simulink model "VINS"  (R2018a)
settings: Solver=FixedStepDiscrete  StartTime=0.0  StopTime=inf  FixedStep=1/Fs  RelTol=1e-3  EnableMultiTasking=on
PreLoadFcn:
  | modelDef = getModelDef(calibrateSFMA);
  | 
  | %imuPar = getImuPar('lmvpUncalibrated');
  | 
  | timeMatchThreshold = 1000;
undefined symbols (not defined in the file or in its folder): beep, dejitter_on, Fs, homogeneous3x4Transform_k_kmin1, imuLocationMm, imuPar, numStates, simData, tstamp_k_us, tstamp_kmin1_us
libraries: simulink x69, dspmtrx3 x35, dspindex x9, vrlib x7, dspstat3 x7, dspinverses x6, dspsigops x5, dspmathops x2, rtwdemowidgets x1, dspfactors x1, simulink_extras x1
(part 3 of 6)

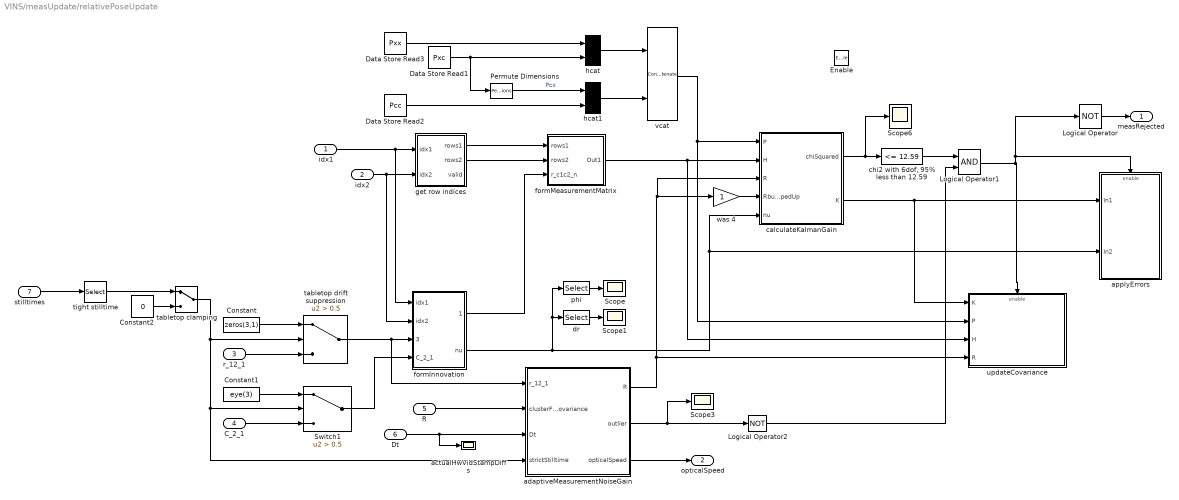
== system VINS/measUpdate/relativePoseUpdate ==
  idx1 : Inport
  idx2 : Inport  Port=2
  r_12_1 : Inport  Port=3
  C_2_1 : Inport  Port=4
  R : Inport  Port=5
  Dt : Inport  Port=6
  stilltimes : Inport  Port=7
  Enable : EnablePort
  Constant : Constant  Value=zeros(3,1)  OutDataTypeStr=Inherit: Inherit via back propagation
  Constant1 : Constant  Value=eye(3)  OutDataTypeStr=Inherit: Inherit via back propagation
  Constant2 : Constant  Value=0
  Data Store Read1 : DataStoreRead  DataStoreName=Pxc
  Data Store Read2 : DataStoreRead  DataStoreName=Pcc
  Data Store Read3 : DataStoreRead  DataStoreName=Pxx
  Logical Operator : Logic  Operator=NOT  Inputs=1  IconShape=distinctive  AllPortsSameDT=off  OutDataTypeStr=boolean
  Logical Operator1 : Logic  AllPortsSameDT=off  OutDataTypeStr=boolean
  Logical Operator2 : Logic  Operator=NOT  Inputs=1  IconShape=distinctive  AllPortsSameDT=off  OutDataTypeStr=boolean
  Permute Dimensions : PermuteDimensions
  Scope{,1,3,6} (4 alike) : Scope
  Switch1 : Switch  Criteria=u2 > Threshold  Threshold=0.5
  actualHwVidStampDiffs : Scope
  adaptiveMeasurementNoiseGain : Subsystem  TreatAsAtomicUnit=on
      settings: RTWSystemCode=Nonreusable function  RTWFcnNameOpts=Use subsystem name
  applyErrors : Subsystem
      settings: RTWSystemCode=Nonreusable function  RTWFcnNameOpts=Use subsystem name
  calculateKalmanGain : MATLAB Function  TreatAsAtomicUnit=on
  "chi2 with 6dof, 95% less than 12.59" : simulink/Logic and Bit Operations/Compare To Constant  relop=<=  const=12.59  OutDataTypeStr=boolean
  dr : Selector  InputPortWidth=6  IndexOptions=Index vector (dialog)  Indices=[4 5 6]  OutputSizes=1
  formInnovation : Subsystem  TreatAsAtomicUnit=on
  formMeasurementMatrix : Subsystem
  get row indices : Subsystem  TreatAsAtomicUnit=on
  hcat : Concatenate  Mode=Multidimensional array  ConcatenateDimension=2
  hcat1 : Concatenate  Mode=Multidimensional array  ConcatenateDimension=2
  phi : Selector  InputPortWidth=6  IndexOptions=Index vector (dialog)  Indices=[1 2 3]  OutputSizes=1
  tabletop clamping : ManualSwitch
  tabletop drift suppression : Switch  Criteria=u2 > Threshold  Threshold=0.5
  tight stilltime : Selector  InputPortWidth=2  IndexOptions=Index vector (dialog)  Indices=1  OutputSizes=1
  updateCovariance : Subsystem
  vcat : Concatenate  Mode=Multidimensional array
  was 4 : Gain  OutDataTypeStr=Inherit: Inherit via back propagation
  measRejected : Outport  OutputWhenDisabled=reset  InitialOutput=0
  opticalSpeed : Outport  Port=2  InitialOutput=100
  wires:
  calculateKalmanGain/2(K) -> updateCovariance/1(K), applyErrors/1(In1)
  vcat/1 -> updateCovariance/2(P), calculateKalmanGain/1(P)
  tabletop drift suppression/1 -> adaptiveMeasurementNoiseGain/1(r_12_1), formInnovation/3(r_c1c2_c1)
  idx1/1 -> formInnovation/1(idx1), get row indices/1(idx1)
  idx2/1 -> formInnovation/2(idx2), get row indices/2(idx2)
  formInnovation/2(nu) -> calculateKalmanGain/5(nu), applyErrors/2(In2), phi/1, dr/1
  formMeasurementMatrix/1(Out1) -> updateCovariance/3(H), calculateKalmanGain/2(H)
  get row indices/1(rows1) -> formMeasurementMatrix/1(rows1)
  get row indices/2(rows2) -> formMeasurementMatrix/2(rows2)
  hcat/1 -> vcat/1
  hcat1/1 -> vcat/2
  Data Store Read3/1 -> hcat/1
  Data Store Read1/1 -> Permute Dimensions/1, hcat/2
  Permute Dimensions/1 -> hcat1/1  "Pcx"
  Data Store Read2/1 -> hcat1/2
  formInnovation/1(r_c1c2_n) -> formMeasurementMatrix/3(r_c1c2_n)
  phi/1 -> Scope/1
  dr/1 -> Scope1/1
  calculateKalmanGain/1(chiSquared) -> "chi2 with 6dof, 95% less than 12.59"/1, Scope6/1
  Logical Operator1/1 -> updateCovariance/Enable, Logical Operator/1, applyErrors/Enable
  Logical Operator/1 -> measRejected/1
  was 4/1 -> calculateKalmanGain/4(RbumpedUp)
  Switch1/1 -> formInnovation/4(C_2_1)
  "chi2 with 6dof, 95% less than 12.59"/1 -> Logical Operator1/1
  R/1 -> adaptiveMeasurementNoiseGain/2(clusterFlowCovariance)
  adaptiveMeasurementNoiseGain/1(R) -> updateCovariance/4(R), calculateKalmanGain/3(R), was 4/1
  adaptiveMeasurementNoiseGain/2(outlier) -> Scope3/1, Logical Operator2/1
  Logical Operator2/1 -> Logical Operator1/2
  Dt/1 -> actualHwVidStampDiffs/1, adaptiveMeasurementNoiseGain/3(Dt)
  C_2_1/1 -> Switch1/3
  r_12_1/1 -> tabletop drift suppression/3
  Constant/1 -> tabletop drift suppression/1
  Constant1/1 -> Switch1/1
  stilltimes/1 -> tight stilltime/1
  tabletop clamping/1 -> tabletop drift suppression/2, adaptiveMeasurementNoiseGain/4(strictStilltime), Switch1/2
  tight stilltime/1 -> tabletop clamping/1
  Constant2/1 -> tabletop clamping/2
  adaptiveMeasurementNoiseGain/3(opticalSpeed) -> opticalSpeed/1

== system VINS/measUpdate/relocalize ==
  note: Absolute Pose Update should trigger relocalization if:
      |      * APU position is > __ cm away from current nav position
      |      * APU heading is > __ mrad away from current naw heading
      |      * current position uncertainty is > __
      |      * current heading uncertainty is > __
      |      * this is the first APU (do we need this?)
  innovation : Inport
  APU : Inport  Port=2
  Bus Selector : BusSelector  OutputSignals=doAbsolutePoseUpdate,r_nb_n,C_b_n
  Subsystem : Subsystem
  reloc : Outport
  wires:
  APU/1 -> Bus Selector/1
  Bus Selector/1 -> Subsystem/Enable  "<doAbsolutePoseUpdate>"
  Bus Selector/2 -> Subsystem/1(r_nc_n)  "<r_nb_n>"
  Bus Selector/3 -> Subsystem/2(<C_b_n>)  "<C_b_n>"
  innovation/1 -> Subsystem/3(innovation)
  Subsystem/1(reloc) -> reloc/1

== system VINS/measUpdate/wipe out delayed states ==
  note: wiping out tstamp_list should be sufficient to cause delayed states in buffers to be ignored
  Enable : EnablePort  ShowOutputPort=on
  Data Store Write5 : DataStoreWrite  DataStoreName=tstamp_list
  Ground : Ground
  setP : Subsystem
  wires:
  Ground/1 -> Data Store Write5/1
  Enable/1 -> setP/Enable

== system VINS/measUpdate/zuptMeasUpdate ==
  stilltime : Inport
  Enable : EnablePort
  0.01s to 10s : Saturate  UpperLimit=10  LowerLimit=0.01
  Constant : Constant  Value=eye(3)  OutDataTypeStr=Inherit: Inherit via back propagation
  Constant1 : Constant  Value=eye(3)  OutDataTypeStr=Inherit: Inherit via back propagation
  Constant2 : Constant  Value=zeros(3,9)  VectorParams1D=off  OutDataTypeStr=Inherit: Inherit via back propagation
  Constant3 : Constant  Value=zeros(3,1)  VectorParams1D=off  OutDataTypeStr=Inherit: Inherit via back propagation
  DT police : Subsystem  TreatAsAtomicUnit=on
  DT police1 : Subsystem  TreatAsAtomicUnit=on
  Data Store Read1 : DataStoreRead  DataStoreName=vnav
  Data Store Read3 : DataStoreRead  DataStoreName=Pxx
  Data Store Write : DataStoreWrite  DataStoreName=Pxx
  Math Function : Math  Operator=reciprocal  SaturateOnIntegerOverflow=on
  Math Function1 : Math  Operator=square  SaturateOnIntegerOverflow=on
  Matrix Concatenate : Concatenate  Mode=Multidimensional array  ConcatenateDimension=2
  Pad : dspsigops/Pad  padAlong=Rows  dimsToPad=1  valSrc=Specify via dialog  padVal=0  spec=Output size  padNumOutRowsSpecMethod=User-specified  numOutRows=1  padNumOutColsSpecMethod=User-specified  numOutCols=modelDef.numStates  isVarDimsMode=off  padBeginning=0  padEnd=0  outSizeMode=User-specified  outSize=1  padSigAt=End  trunc_flag=None  roundingMode=Floor  overflowMode=off  truncOrWrapMode=Truncate  wrap_flag=None
      settings: SourceProductName=DSP System Toolbox  SourceProductBaseCode=DS
  Product1 : Product  Multiplication=Matrix(*)
  Product2 : Product
  Saturation : Saturate  UpperLimit=100  LowerLimit=0.1
  Scope : Scope
  Scope1 : Scope
  Selector : Selector  InputPortWidth=2  IndexOptions=Index vector (dialog)  Indices=2  OutputSizes=1
  Sum1 : Sum  Inputs=|+-
  applyErrors : Subsystem
  calculateKalmanGain : MATLAB Function  TreatAsAtomicUnit=on
  josephCovarianceUpdate : MATLAB Function  TreatAsAtomicUnit=on
  wires:
  Constant3/1 -> Sum1/2
  Data Store Read1/1 -> Sum1/1
  0.01s to 10s/1 -> Math Function/1
  Constant1/1 -> Matrix Concatenate/2
  Constant2/1 -> Matrix Concatenate/1
  Sum1/1 -> Product1/2, Scope1/1  "nu = dv = vhat - vtrue"
  josephCovarianceUpdate/1(Pplus) -> Data Store Write/1
  Matrix Concatenate/1 -> Pad/1
  Data Store Read3/1 -> josephCovarianceUpdate/1(P), calculateKalmanGain/1(P)
  Product2/1 -> DT police1/1(In1), josephCovarianceUpdate/4(R), calculateKalmanGain/3(R)
  Product1/1 -> applyErrors/1(errorStateEstimates)  "errors"
  Constant/1 -> Product2/1
  Math Function/1 -> Saturation/1
  Saturation/1 -> Math Function1/1, Scope/1
  stilltime/1 -> Selector/1
  Math Function1/1 -> Product2/2
  Pad/1 -> DT police/1(In1), josephCovarianceUpdate/3(H), calculateKalmanGain/2(H)
  calculateKalmanGain/2(K) -> josephCovarianceUpdate/2(K), Product1/1
  Selector/1 -> 0.01s to 10s/1

== system VINS/reportOutputs/dejitter ==
  note: Velocity of corrections should be limited to 10% of the
      | optical velocity when confident optical velocity exists.
      |
      | However, to prevent unbounded drift,  increase the correction factor if the error gets very large.
  r_jit : Inport
  v : Inport  Port=2
  opticalSpeed : Inport  Port=3
  Dt : Inport  Port=4
  reloc : Inport  Port=5
  1-D Lookup Table : Lookup_n-D  NumberOfTableDimensions=1  BreakpointsForDimension1="[0  0.005 0.01 0.02 0.03 0.04]"  Table="[0    0.02   0.08    0.2       1      1]"  InternalRulePriority=Speed  RndMeth=Simplest  InputSameDT=on
  1-D Lookup Table1 : Lookup_n-D  Commented=on  NumberOfTableDimensions=1  BreakpointsForDimension1="[0  0.05 0.1 0.2 0.3 0.4]"  Table="[0.002    0.02   0.08    0.2       1      1]*0.1"  InternalRulePriority=Speed  RndMeth=Simplest  InputSameDT=on
  Gain : Gain  Gain=1/2
  Gain1 : Gain  Gain=0.1
  Math Function : Math  Operator=square  SaturateOnIntegerOverflow=on
  Math Function1 : Math  Operator=square  SaturateOnIntegerOverflow=on
  MinMax : MinMax  Function=max  Inputs=2
  Product : Product
  Product1 : Product
  Product2 : Product
  Scope1 : Scope  NumInputPorts=2
  Scope2 : Scope
  Scope3 : Scope
  Sqrt : Sqrt  SaturateOnIntegerOverflow=on
  Sqrt1 : Sqrt  SaturateOnIntegerOverflow=on
  Sum : Sum  Inputs=|++
  Sum1 : Sum
  Sum2 : Sum  Inputs=|+-
  Sum3 : Sum  Inputs=|++
  Sum4 : Sum  Inputs=+
  Sum5 : Sum  Inputs=+
  midpoint velocity : Delay  DelayLength=1  InitialConditionSource=Input port
      settings: InputPortMap=u0,p4
  position integrator : Delay  DelayLength=1  InitialConditionSource=Input port  ExternalReset=Level
      settings: InputPortMap=u0,r5,p4
  r_clean : Outport
  wires:
  position integrator/1 -> Sum1/2
  r_jit/1 -> Sum2/1, position integrator/3  "measPos"
  v/1 -> Sum/1, midpoint velocity/2, midpoint velocity/1
  midpoint velocity/1 -> Sum/2
  Sum/1 -> Gain/1
  Gain/1 -> Product/1, Math Function1/1
  Product/1 -> Sum1/1
  Sum1/1 -> Sum3/2, Sum2/2  "predPos"
  Sum2/1 -> Math Function/1, Product1/2  "innov"
  Product1/1 -> Sum3/1
  Sum3/1 -> position integrator/1, r_clean/1
  Math Function/1 -> Sum4/1
  Sum4/1 -> Sqrt/1
  Sqrt/1 -> 1-D Lookup Table/1, Product2/2  "needed delta_r"
  MinMax/1 -> Product1/1, Scope3/1  "jitter fraction"
  Sum5/1 -> Sqrt1/1
  Math Function1/1 -> Sum5/1
  Sqrt1/1 -> Scope1/2, 1-D Lookup Table1/1, Gain1/1  "INS speed"
  reloc/1 -> position integrator/2
  Gain1/1 -> MinMax/1
  Product2/1 -> Scope2/1, MinMax/2
  1-D Lookup Table/1 -> Product2/1
  Dt/1 -> Product/2
  opticalSpeed/1 -> Scope1/1

== system VINS/reportOutputs/updateDistTravelled ==
  pos : Inport
  Compare To Constant : simulink/Logic and Bit Operations/Compare To Constant  relop=>=  const=0.003  OutDataTypeStr=boolean
  Compare To Zero : simulink/Logic and Bit Operations/Compare To Zero  relop===  OutDataTypeStr=boolean
  Data Store Read : DataStoreRead  DataStoreName=distTravelled
  Logical Operator : Logic  Operator=OR  AllPortsSameDT=off  OutDataTypeStr=boolean
  Math Function : Math  Operator=square  SaturateOnIntegerOverflow=on
  Sqrt : Sqrt  SaturateOnIntegerOverflow=on
  Sum2 : Sum  Inputs=|+-
  Sum4 : Sum  Inputs=+
  Unit Delay : UnitDelay  SampleTime=-1
  increment distTravelled : Subsystem  TreatAsAtomicUnit=on
  latch : Subsystem  TreatAsAtomicUnit=on
  reset occured : simulink/Logic and Bit Operations/Detect Rise Positive  vinit=0  OutDataTypeStr=boolean
  distTravelled : Outport
  wires:
  pos/1 -> Sum2/1, latch/1(In1)  "measPos"
  latch/1(Out1) -> Sum2/2  "predPos"
  Sum2/1 -> Math Function/1  "innov"
  Math Function/1 -> Sum4/1
  Sum4/1 -> Sqrt/1
  Sqrt/1 -> increment distTravelled/1(deltaPos), Compare To Constant/1  "position change"
  Data Store Read/1 -> Compare To Zero/1
  Compare To Zero/1 -> reset occured/1
  reset occured/1 -> Logical Operator/2
  Compare To Constant/1 -> Unit Delay/1, increment distTravelled/Enable
  increment distTravelled/1(distTravelled) -> distTravelled/1
  Logical Operator/1 -> latch/Enable
  Unit Delay/1 -> Logical Operator/1

== system VINS/sensorCompensation/DT police ==
  In1 : Inport
  Data Store Read : DataStoreRead  DataStoreName=DataTypeRef
  Data Type Duplicate : DataTypeDuplicate
  wires:
  Data Store Read/1 -> Data Type Duplicate/1
  In1/1 -> Data Type Duplicate/2

== system VINS/sensorCompensation/DT police1 ==
  In1 : Inport
  Data Store Read : DataStoreRead  DataStoreName=DataTypeRef
  Data Type Duplicate : DataTypeDuplicate
  wires:
  In1/1 -> Data Type Duplicate/2
  Data Store Read/1 -> Data Type Duplicate/1

== system VINS/sensorCompensation/detectAccelSaturation ==
  In1 : Inport
  Abs : Abs
  Abs1 : Abs
  Abs2 : Abs
  Compare To Constant : simulink/Logic and Bit Operations/Compare To Constant  relop=>  const=39  OutDataTypeStr=boolean
  Compare To Constant1 : simulink/Logic and Bit Operations/Compare To Constant  relop=<  const=0.002  OutDataTypeStr=boolean
  Compare To Constant2 : simulink/Logic and Bit Operations/Compare To Constant  relop=<  const=0.002  OutDataTypeStr=boolean
  Logical Operator : Logic  Inputs=3  AllPortsSameDT=off  OutDataTypeStr=boolean
  Logical Operator1 : Logic  Operator=OR  Inputs=1  AllPortsSameDT=off  OutDataTypeStr=boolean
  Logical Operator2 : Logic  AllPortsSameDT=off  OutDataTypeStr=boolean
  Logical Operator3 : Logic  AllPortsSameDT=off  OutDataTypeStr=boolean
  Scope : Scope
  Scope1 : Scope
  Scope2 : Scope
  Sum1 : Sum  Inputs=+-|
  Sum2 : Sum  Inputs=+-|
  Unit Delay{,1..3} (4 alike) : UnitDelay  SampleTime=-1
  set 0x01 bit : Subsystem  TreatAsAtomicUnit=on
  wires:
  Logical Operator/1 -> Scope/1, Logical Operator3/1
  Unit Delay1/1 -> Logical Operator/3
  Unit Delay/1 -> Logical Operator/2, Unit Delay1/1
  Compare To Constant/1 -> Logical Operator/1, Unit Delay/1
  Abs/1 -> Compare To Constant/1
  In1/1 -> Sum1/2, Unit Delay2/1, Abs/1
  Sum2/1 -> Abs1/1
  Sum1/1 -> Abs2/1
  Abs1/1 -> Compare To Constant1/1
  Abs2/1 -> Compare To Constant2/1
  Logical Operator2/1 -> Scope1/1, Logical Operator3/2
  Logical Operator3/1 -> Logical Operator1/1
  Logical Operator1/1 -> Scope2/1, set 0x01 bit/Enable
  Unit Delay2/1 -> Unit Delay3/1, Sum2/2, Sum1/1
  Unit Delay3/1 -> Sum2/1
  Compare To Constant1/1 -> Logical Operator2/1
  Compare To Constant2/1 -> Logical Operator2/2

== system VINS/sensorCompensation/detectGyroSaturation ==
  In1 : Inport
  Abs : Abs
  Compare To Constant : simulink/Logic and Bit Operations/Compare To Constant  relop=>  const=1900*pi/180  OutDataTypeStr=boolean
  Logical Operator : Logic  Inputs=3  AllPortsSameDT=off  OutDataTypeStr=boolean
  Logical Operator1 : Logic  Operator=OR  Inputs=1  AllPortsSameDT=off  OutDataTypeStr=boolean
  Unit Delay : UnitDelay  SampleTime=-1
  Unit Delay1 : UnitDelay  SampleTime=-1
  set 0x02 bit : Subsystem  TreatAsAtomicUnit=on
  wires:
  In1/1 -> Abs/1
  Abs/1 -> Compare To Constant/1
  Compare To Constant/1 -> Unit Delay/1, Logical Operator/1
  Unit Delay/1 -> Unit Delay1/1, Logical Operator/2
  Unit Delay1/1 -> Logical Operator/3
  Logical Operator/1 -> Logical Operator1/1
  Logical Operator1/1 -> set 0x02 bit/Enable

== system VINS/sensorCompensation/set 0x04 bit ==
  Enable : EnablePort
  Assertion : Assertion  StopWhenAssertionFail=off
  Bit Set : simulink/Logic and Bit Operations/Bit Set  iBit=2
      settings: SourceProductName=Simulink  SourceProductBaseCode=SL
  Constant : Constant  Value=false
  Data Store Read : DataStoreRead  DataStoreName=errorBitfield
  Data Store Write : DataStoreWrite  DataStoreName=errorBitfield
  wires:
  Data Store Read/1 -> Bit Set/1
  Bit Set/1 -> Data Store Write/1
  Constant/1 -> Assertion/1

== system VINS/stilltimes/DT police ==
  In1 : Inport
  Data Store Read : DataStoreRead  DataStoreName=DataTypeRef
  Data Type Duplicate : DataTypeDuplicate
  wires:
  Data Store Read/1 -> Data Type Duplicate/1
  In1/1 -> Data Type Duplicate/2

== system VINS/stilltimes/DT police1 ==
  In1 : Inport
  Data Store Read : DataStoreRead  DataStoreName=DataTypeRef
  Data Type Duplicate : DataTypeDuplicate
  wires:
  In1/1 -> Data Type Duplicate/2
  Data Store Read/1 -> Data Type Duplicate/1

== system VINS/uncomment and set zero noise for verification/compare  timestamps ==
  t1_meas : Inport
  t1_pred : Inport  Port=2
  t2_meas : Inport  Port=3
  t2_pred : Inport  Port=4
  Enable : EnablePort
  Assertion : Assertion  Commented=on
  Assertion1 : Assertion  Commented=on
  Compare To Constant : simulink/Logic and Bit Operations/Compare To Constant  relop=<=  const=3.0  OutDataTypeStr=boolean
  Compare To Constant1 : simulink/Logic and Bit Operations/Compare To Constant  relop=<=  const=3.0  OutDataTypeStr=boolean
  Scope : Scope
  Scope1 : Scope
  Scope2 : Scope
  Sum : Sum  Inputs=|+-
  Sum1 : Sum  Inputs=|+-
  Sum2 : Sum  Inputs=|+-
  Unit Delay : UnitDelay  SampleTime=-1
  wires:
  Sum/1 -> Compare To Constant/1, Scope/1
  t1_meas/1 -> Sum2/1, Sum/1
  t2_meas/1 -> Unit Delay/1, Sum1/1
  Sum1/1 -> Compare To Constant1/1, Scope1/1
  t1_pred/1 -> Sum/2
  t2_pred/1 -> Sum1/2
  Compare To Constant/1 -> Assertion/1
  Compare To Constant1/1 -> Assertion1/1
  Unit Delay/1 -> Sum2/2
  Sum2/1 -> Scope2/1

== system VINS/uncomment and set zero noise for verification/initialize H ==
  Enable : EnablePort
  Constant : Constant  Value=[0 0 0 1]  VectorParams1D=off  OutDataTypeStr=Inherit: Inherit via back propagation
  Constant9 : Constant  Value=imuLocationMm  OutDataTypeStr=Inherit: Inherit via back propagation
  Data Store Read : DataStoreRead  DataStoreName=Cbn
  Data Store Read1 : DataStoreRead  DataStoreName=rnav
  Data Store Write : DataStoreWrite  DataStoreName=H
  Gain : Gain  Gain=1/1000
  Matrix Concatenate : Concatenate  Mode=Multidimensional array  ConcatenateDimension=2
  Matrix Concatenate1 : Concatenate  Mode=Multidimensional array
  Matrix Multiply : Product  Multiplication=Matrix(*)
  Sum : Sum  Inputs=-+|
  wires:
  Constant/1 -> Matrix Concatenate1/2
  Sum/1 -> Matrix Concatenate/2  "r_nc_n"
  Matrix Concatenate/1 -> Matrix Concatenate1/1
  Matrix Concatenate1/1 -> Data Store Write/1
  Data Store Read1/1 -> Sum/2  "r_nb_n"
  Constant9/1 -> Gain/1
  Matrix Multiply/1 -> Sum/1  "r_cb_n"
  Data Store Read/1 -> Matrix Multiply/1, Matrix Concatenate/1  "Ccn = Cbn"
  Gain/1 -> Matrix Multiply/2  "r_cb_c"

== system VINS/uncomment and set zero noise for verification/latch ==
  r_12_1 : Inport
  C_2_1 : Inport  Port=2
  t1 : Inport  Port=3
  t2 : Inport  Port=4
  delayFrames : Inport  Port=5
  Enable : EnablePort
  Delay{,1..3} (4 alike) : Delay  DelayLengthSource=Input port
      settings: InputPortMap=u0,p1
  r21 : Outport
  C21 : Outport  Port=2
  tout1 : Outport  Port=3
  tout2 : Outport  Port=4
  wires:
  r_12_1/1 -> Delay/1
  C_2_1/1 -> Delay1/1
  t1/1 -> Delay2/1
  t2/1 -> Delay3/1
  Delay/1 -> r21/1
  Delay1/1 -> C21/1
  Delay2/1 -> tout1/1
  Delay3/1 -> tout2/1
  delayFrames/1 -> Delay3/2, Delay2/2, Delay1/2, Delay/2

== system VINS/uncomment and set zero noise for verification/plot errors ==
  dr_meas : Inport
  C21_meas : Inport  Port=2
  dr_pred : Inport  Port=3
  C21_pred : Inport  Port=4
  Enable : EnablePort
  Cumulative Sum : dspmathops/Cumulative Sum  dim=Channels (running sum)  reset_popup=None  roundingMode=Floor  overflowMode=off  outputDataTypeStr=Inherit: Same as accumulator  outputMin=[]  outputMax=[]  outputLastDataTypeStr=Inherit: Same as accumulator
      settings: SourceProductName=DSP System Toolbox
  Cumulative Sum1 : dspmathops/Cumulative Sum  dim=Channels (running sum)  reset_popup=None  roundingMode=Floor  overflowMode=off  outputDataTypeStr=Inherit: Same as accumulator  outputMin=[]  outputMax=[]  outputLastDataTypeStr=Inherit: Same as accumulator
      settings: SourceProductName=DSP System Toolbox
  MATLAB Function1 : MATLAB Function  TreatAsAtomicUnit=on
  MATLAB Function2 : MATLAB Function  TreatAsAtomicUnit=on
  MATLAB Function3 : MATLAB Function  TreatAsAtomicUnit=on
  Matrix Multiply : Product  Multiplication=Matrix(*)
  Permute Dimensions : PermuteDimensions
  Reshape : Reshape
  Scope{,1..2,5..6} (5 alike) : Scope
  Scope3 : Scope  NumInputPorts=2
  Scope4 : Scope  NumInputPorts=2
  Sum : Sum  Inputs=|+-
  det3x3 : Fcn  Expr=|
      | u(1)*
      | (u(5)*u(9) - u(8)*u(6)
      | ) - u(4)*
      | (u(2)*
      | u(9) - u(8)*u(3)
      | ) + u(7)*
      | (u(2)*u(6) - u(5)*u(3)
      | )
  deul_meas : Outport
  deul_pred : Outport  Port=2
  drmeas : Outport  Port=3
  drpred : Outport  Port=4
  wires:
  dr_meas/1 -> drmeas/1, Scope4/1, Cumulative Sum/1, Sum/1
  Sum/1 -> Scope/1
  Permute Dimensions/1 -> Matrix Multiply/2
  Matrix Multiply/1 -> MATLAB Function3/1(Cbn)
  MATLAB Function3/1(eul) -> Scope1/1
  MATLAB Function1/1(eul) -> Cumulative Sum1/1, deul_meas/1, Scope3/1
  MATLAB Function2/1(eul) -> deul_pred/1, Scope3/2
  det3x3/1 -> Scope5/1
  Reshape/1 -> det3x3/1
  C21_meas/1 -> MATLAB Function1/1(Cbn), Matrix Multiply/1, Reshape/1
  C21_pred/1 -> MATLAB Function2/1(Cbn), Permute Dimensions/1
  dr_pred/1 -> Scope4/2, drpred/1, Sum/2
  Cumulative Sum/1 -> Scope2/1  "translation cumsum"
  Cumulative Sum1/1 -> Scope6/1  "rotation cumsum"

== system VINS/uncomment and set zero noise for verification/update pure optical pose ==
  r_2_1 : Inport
  C_2_1 : Inport  Port=2
  Enable : EnablePort
  Constant : Constant  Value=[0 0 0 1]  VectorParams1D=off  OutDataTypeStr=Inherit: Inherit via back propagation
  DT police : Subsystem  TreatAsAtomicUnit=on
  Data Store Read : DataStoreRead  DataStoreName=H
  Data Store Read1 : DataStoreRead  DataStoreName=INITIALIZED
  Data Store Write : DataStoreWrite  DataStoreName=H
  Detect Rise Positive : simulink/Logic and Bit Operations/Detect Rise Positive  vinit=0  OutDataTypeStr=boolean
  MATLAB Function1 : MATLAB Function  TreatAsAtomicUnit=on
  Matrix Concatenate : Concatenate  Mode=Multidimensional array  ConcatenateDimension=2
  Matrix Concatenate1 : Concatenate  Mode=Multidimensional array
  Matrix Multiply : Product  Multiplication=Matrix(*)
  extract C : dspmtrx3/Submatrix  RowSpan=Range of rows  RowStartMode=First  RowStartIndex=1  RowEndMode=Index  RowEndIndex=3  ColSpan=Range of columns  ColStartMode=First  ColStartIndex=1  ColEndMode=Index  ColEndIndex=3
  extract r : dspmtrx3/Submatrix  RowSpan=Range of rows  RowStartMode=First  RowStartIndex=1  RowEndMode=Index  RowEndIndex=3  ColSpan=One column  ColStartMode=Last  ColStartIndex=1  ColEndMode=Last  ColEndIndex=1
  initialize H : Subsystem  TreatAsAtomicUnit=on
  r : Outport
  eulers : Outport  Port=2
  wires:
  C_2_1/1 -> Matrix Concatenate/1
  r_2_1/1 -> Matrix Concatenate/2
  Matrix Concatenate/1 -> Matrix Concatenate1/1
  Constant/1 -> Matrix Concatenate1/2
  Data Store Read/1 -> Matrix Multiply/1
  Matrix Concatenate1/1 -> Matrix Multiply/2
  Matrix Multiply/1 -> extract r/1, Data Store Write/1, DT police/1(In1), extract C/1
  extract r/1 -> r/1
  extract C/1 -> MATLAB Function1/1(Cbn)
  MATLAB Function1/1(eul) -> eulers/1
  Data Store Read1/1 -> Detect Rise Positive/1
  Detect Rise Positive/1 -> initialize H/Enable

== system VINS/cameraRelativePosePrediction/localIns/DT police ==
  In1 : Inport
  Data Store Read : DataStoreRead  DataStoreName=DataTypeRef
  Data Type Duplicate : DataTypeDuplicate
  wires:
  Data Store Read/1 -> Data Type Duplicate/1
  In1/1 -> Data Type Duplicate/2

== system VINS/cameraRelativePosePrediction/localIns/cloneGlobalInsStates AFTER the update ==
  Enable : EnablePort
  Data Store Read : DataStoreRead  DataStoreName=Cbn
  Data Store Read1 : DataStoreRead  DataStoreName=vnav
  Data Store Read2 : DataStoreRead  DataStoreName=rnav
  Data Store Write : DataStoreWrite  DataStoreName=CbnLocal
  Data Store Write1 : DataStoreWrite  DataStoreName=vnavLocal
  Data Store Write2 : DataStoreWrite  DataStoreName=rnavLocal
  Unit Delay : UnitDelay  SampleTime=-1
  Unit Delay1 : UnitDelay  SampleTime=-1
  prev_r : Outport
  prev_C : Outport  Port=2
  wires:
  Data Store Read/1 -> Unit Delay1/1, Data Store Write/1
  Data Store Read1/1 -> Data Store Write1/1
  Data Store Read2/1 -> Unit Delay/1, Data Store Write2/1
  Unit Delay/1 -> prev_r/1
  Unit Delay1/1 -> prev_C/1

== system VINS/initStatesCovariances/initialize r_bc_b/DT police ==
  In1 : Inport
  Data Store Read : DataStoreRead  DataStoreName=DataTypeRef
  Data Type Duplicate : DataTypeDuplicate
  wires:
  Data Store Read/1 -> Data Type Duplicate/1
  In1/1 -> Data Type Duplicate/2

== system VINS/initStatesCovariances/pefectInit (only for development testing)/DT convert1 ==
  In1 : Inport
  Data Store Read : DataStoreRead  DataStoreName=DataTypeRef
  Data Type Conversion Inherited : simulink/Signal Attributes/Data Type Conversion Inherited  ConvertRealWorld=Real World Value  DoSatur=off
      settings: SourceProductName=Simulink  SourceProductBaseCode=SL
  Out1 : Outport
  wires:
  In1/1 -> Data Type Conversion Inherited/2
  Data Store Read/1 -> Data Type Conversion Inherited/1
  Data Type Conversion Inherited/1 -> Out1/1

== system VINS/initStatesCovariances/pefectInit (only for development testing)/DT convert2 ==
  In1 : Inport
  Data Store Read : DataStoreRead  DataStoreName=DataTypeRef
  Data Type Conversion Inherited : simulink/Signal Attributes/Data Type Conversion Inherited  ConvertRealWorld=Real World Value  DoSatur=off
      settings: SourceProductName=Simulink  SourceProductBaseCode=SL
  Out1 : Outport
  wires:
  Data Type Conversion Inherited/1 -> Out1/1
  Data Store Read/1 -> Data Type Conversion Inherited/1
  In1/1 -> Data Type Conversion Inherited/2

== system VINS/initStatesCovariances/pefectInit (only for development testing)/DT convert3 ==
  In1 : Inport
  Data Store Read : DataStoreRead  DataStoreName=DataTypeRef
  Data Type Conversion Inherited : simulink/Signal Attributes/Data Type Conversion Inherited  ConvertRealWorld=Real World Value  DoSatur=off
      settings: SourceProductName=Simulink  SourceProductBaseCode=SL
  Out1 : Outport
  wires:
  In1/1 -> Data Type Conversion Inherited/2
  Data Store Read/1 -> Data Type Conversion Inherited/1
  Data Type Conversion Inherited/1 -> Out1/1

== system VINS/initStatesCovariances/pefectInit (only for development testing)/DT convert4 ==
  In1 : Inport
  Data Store Read : DataStoreRead  DataStoreName=DataTypeRef
  Data Type Conversion Inherited : simulink/Signal Attributes/Data Type Conversion Inherited  ConvertRealWorld=Real World Value  DoSatur=off
      settings: SourceProductName=Simulink  SourceProductBaseCode=SL
  Out1 : Outport
  wires:
  Data Type Conversion Inherited/1 -> Out1/1
  Data Store Read/1 -> Data Type Conversion Inherited/1
  In1/1 -> Data Type Conversion Inherited/2

== system VINS/initStatesCovariances/pefectInit (only for development testing)/DT police ==
  In1 : Inport
  Data Store Read : DataStoreRead  DataStoreName=DataTypeRef
  Data Type Duplicate : DataTypeDuplicate
  wires:
  Data Store Read/1 -> Data Type Duplicate/1
  In1/1 -> Data Type Duplicate/2

== system VINS/initStatesCovariances/pefectInit (only for development testing)/DT police3 ==
  In1 : Inport
  Data Store Read : DataStoreRead  DataStoreName=DataTypeRef
  Data Type Duplicate : DataTypeDuplicate
  wires:
  Data Store Read/1 -> Data Type Duplicate/1
  In1/1 -> Data Type Duplicate/2

== system VINS/initStatesCovariances/realInit/calcCbn ==
  f^b : Inport
  Enable : EnablePort  ShowOutputPort=on
  Bus Selector : BusSelector  OutputSignals=Cbn
  Constant : Constant  Value=[1 0 0]  VectorParams1D=off  OutDataTypeStr=Inherit: Inherit via back propagation
  Constant1 : Constant  Value=eye(3)  OutDataTypeStr=Inherit: Inherit via back propagation
  Constant2 : Constant  Value=0  OutDataTypeStr=Inherit: Inherit via back propagation
  Constant3 : Constant  OutDataTypeStr=Inherit: Inherit via back propagation
  Cross Product : vrlib/Utilities/Cross Product
      settings: SourceProductBaseCode=VR
  Cross Product1 : vrlib/Utilities/Cross Product
      settings: SourceProductBaseCode=VR
  DT convert : Subsystem
  DT convert1 : Subsystem
  DT police : Subsystem  TreatAsAtomicUnit=on
  DT police2 : Subsystem  TreatAsAtomicUnit=on
  Data Store Read1 : DataStoreRead  DataStoreName=truthTraj  DataStoreElements=truthTraj
  Environment Controller : simulink/Signal Routing/Environment Controller
      settings: SourceProductName=Simulink  SourceProductBaseCode=SL
  Gain : Gain  Gain=-1
  Gain1 : Gain  Gain=-1
  MATLAB Function3 : MATLAB Function  TreatAsAtomicUnit=on
  Matrix Concatenate : Concatenate  NumInputs=3  Mode=Multidimensional array
  Matrix Multiply : Product  Multiplication=Matrix(*)
  Mux : Mux  Inputs=9
  Normalize Vector : vrlib/Utilities/Normalize Vector  maxzero=0
      settings: SourceProductName=Simulink 3D Animation  SourceProductBaseCode=VR
  Normalize Vector1 : vrlib/Utilities/Normalize Vector  maxzero=0
      settings: SourceProductName=Simulink 3D Animation  SourceProductBaseCode=VR
  Normalize Vector2 : vrlib/Utilities/Normalize Vector  maxzero=0
      settings: SourceProductName=Simulink 3D Animation  SourceProductBaseCode=VR
  Reshape : Reshape  OutputDimensionality=Customize  OutputDimensions=[3,3]
  Reshape1 : Reshape  OutputDimensionality=Row vector (2-D)  OutputDimensions=[3,3]
  Selector : Selector  InputPortWidth=3  IndexOptions=Index vector (dialog)  Indices=3  OutputSizes=1
  Trigonometric Function : Trigonometry
  Trigonometric Function1 : Trigonometry  Operator=cos
  yaw only rot matrix : Reshape  OutputDimensionality=Customize  OutputDimensions=[3,3]
  Out1 : Outport  OutputWhenDisabled=reset  InitialOutput=false
  Cbn : Outport  Port=2
  wires:
  Enable/1 -> Out1/1
  Matrix Concatenate/1 -> DT convert1/1(In1)  "yaw zero rot matrix"
  Normalize Vector2/1 -> Matrix Concatenate/3
  Normalize Vector1/1 -> Matrix Concatenate/2
  Normalize Vector/1 -> Matrix Concatenate/1
  Cross Product1/1 -> Normalize Vector/1  "north^b"
  Cross Product/1 -> Cross Product1/1, Normalize Vector1/1  "east^b"
  Gain/1 -> Cross Product/1, Cross Product1/2, Normalize Vector2/1  "down^b"
  f^b/1 -> Reshape1/1  "up"
  Bus Selector/1 -> DT convert/1(In1)  "<Cbn>"
  Reshape/1 -> MATLAB Function3/1(Cbn)
  Data Store Read1/1 -> Bus Selector/1
  Constant/1 -> DT police2/1(In1), Cross Product/2
  MATLAB Function3/1(eul) -> Selector/1
  Selector/1 -> Trigonometric Function/1, Trigonometric Function1/1
  yaw only rot matrix/1 -> Environment Controller/1
  Constant1/1 -> Environment Controller/2
  Environment Controller/1 -> DT police/1(In1), Matrix Multiply/1
  Matrix Multiply/1 -> Cbn/1
  Trigonometric Function1/1 -> Mux/5, Mux/1
  Trigonometric Function/1 -> Mux/2, Gain1/1
  Constant2/1 -> Mux/8, Mux/7, Mux/6, Mux/3
  Gain1/1 -> Mux/4
  Constant3/1 -> Mux/9
  Mux/1 -> yaw only rot matrix/1
  Reshape1/1 -> Gain/1
  DT convert/1(Out1) -> Reshape/1
  DT convert1/1(Out1) -> Matrix Multiply/2

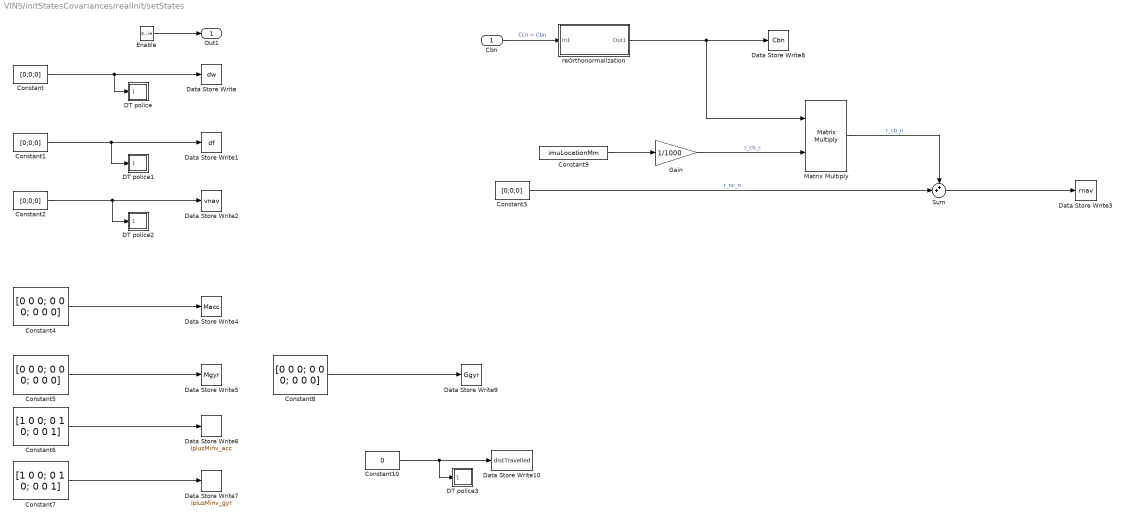
== system VINS/initStatesCovariances/realInit/setStates ==
  Cbn : Inport
  Enable : EnablePort  ShowOutputPort=on
  Constant{,1..3} (4 alike) : Constant  Value=[0;0;0]  OutDataTypeStr=Inherit: Inherit via back propagation
  Constant10 : Constant  Value=0  OutDataTypeStr=Inherit: Inherit via back propagation
  Constant4 : Constant  Value=[0 0 0; 0 0 0; 0 0 0]  VectorParams1D=off  OutDataTypeStr=Inherit: Inherit via back propagation
  Constant5 : Constant  Value=[0 0 0; 0 0 0; 0 0 0]  VectorParams1D=off  OutDataTypeStr=Inherit: Inherit via back propagation
  Constant6 : Constant  Value=[1 0 0; 0 1 0; 0 0 1]  VectorParams1D=off  OutDataTypeStr=Inherit: Inherit via back propagation
  Constant7 : Constant  Value=[1 0 0; 0 1 0; 0 0 1]  VectorParams1D=off  OutDataTypeStr=Inherit: Inherit via back propagation
  Constant8 : Constant  Value=[0 0 0; 0 0 0; 0 0 0]  VectorParams1D=off  OutDataTypeStr=Inherit: Inherit via back propagation
  Constant9 : Constant  Value=imuLocationMm  OutDataTypeStr=Inherit: Inherit via back propagation
  DT police : Subsystem  TreatAsAtomicUnit=on
  DT police1 : Subsystem  TreatAsAtomicUnit=on
  DT police2 : Subsystem  TreatAsAtomicUnit=on
  DT police3 : Subsystem  TreatAsAtomicUnit=on
  Data Store Write : DataStoreWrite  DataStoreName=dw
  Data Store Write1 : DataStoreWrite  DataStoreName=df
  Data Store Write10 : DataStoreWrite  DataStoreName=distTravelled
  Data Store Write2 : DataStoreWrite  DataStoreName=vnav
  Data Store Write3 : DataStoreWrite  DataStoreName=rnav
  Data Store Write4 : DataStoreWrite  DataStoreName=Macc
  Data Store Write5 : DataStoreWrite  DataStoreName=Mgyr
  Data Store Write6 : DataStoreWrite  DataStoreName=IplusMinv_acc
  Data Store Write7 : DataStoreWrite  DataStoreName=IplusMinv_gyr
  Data Store Write8 : DataStoreWrite  DataStoreName=Cbn
  Data Store Write9 : DataStoreWrite  DataStoreName=Ggyr
  Gain : Gain  Gain=1/1000
  Matrix Multiply : Product  Multiplication=Matrix(*)
  Sum : Sum  Inputs=++|
  reOrthonormalization : Subsystem  TreatAsAtomicUnit=on
  Out1 : Outport  OutputWhenDisabled=reset  InitialOutput=false
  wires:
  Constant8/1 -> Data Store Write9/1
  Enable/1 -> Out1/1
  Constant7/1 -> Data Store Write7/1
  Constant6/1 -> Data Store Write6/1
  Constant5/1 -> Data Store Write5/1
  Constant4/1 -> Data Store Write4/1
  Constant2/1 -> DT police2/1(In1), Data Store Write2/1
  Constant1/1 -> DT police1/1(In1), Data Store Write1/1
  Constant/1 -> DT police/1(In1), Data Store Write/1
  Sum/1 -> Data Store Write3/1
  Matrix Multiply/1 -> Sum/1  "r_cb_n"
  Cbn/1 -> reOrthonormalization/1(In1)  "Ccn = Cbn"
  Constant9/1 -> Gain/1
  Constant3/1 -> Sum/2  "r_nc_n"
  Constant10/1 -> DT police3/1(In1), Data Store Write10/1
  Gain/1 -> Matrix Multiply/2  "r_cb_c"
  reOrthonormalization/1(Out1) -> Matrix Multiply/1, Data Store Write8/1

== system VINS/initStatesCovariances/setP/DT police1 ==
  In1 : Inport
  Data Store Read : DataStoreRead  DataStoreName=DataTypeRef
  Data Type Duplicate : DataTypeDuplicate
  wires:
  Data Store Read/1 -> Data Type Duplicate/1
  In1/1 -> Data Type Duplicate/2

== system VINS/initStatesCovariances/setP/DT police2 ==
  In1 : Inport
  Data Store Read : DataStoreRead  DataStoreName=DataTypeRef
  Data Type Duplicate : DataTypeDuplicate
  wires:
  In1/1 -> Data Type Duplicate/2
  Data Store Read/1 -> Data Type Duplicate/1

== system VINS/initStatesCovariances/setP/DT police3 ==
  In1 : Inport
  Data Store Read : DataStoreRead  DataStoreName=DataTypeRef
  Data Type Duplicate : DataTypeDuplicate
  wires:
  Data Store Read/1 -> Data Type Duplicate/1
  In1/1 -> Data Type Duplicate/2

== system VINS/measUpdate/absolutePoseUpdate/DT police ==
  In1 : Inport
  Data Store Read : DataStoreRead  DataStoreName=DataTypeRef
  Data Type Duplicate : DataTypeDuplicate
  wires:
  Data Store Read/1 -> Data Type Duplicate/1
  In1/1 -> Data Type Duplicate/2

== system VINS/measUpdate/absolutePoseUpdate/applyErrors ==
  errors : Inport
  Enable : EnablePort
  Data Store Read : DataStoreRead  DataStoreName=C_b_n_list
  Data Store Read1 : DataStoreRead  DataStoreName=r_b_n_list
  Data Store Write : DataStoreWrite  DataStoreName=C_b_n_list
  Data Store Write1 : DataStoreWrite  DataStoreName=r_b_n_list
  For Each Subsystem : Subsystem  TreatAsAtomicUnit=on
  Pad : dspsigops/Pad  padAlong=Columns  dimsToPad=1  valSrc=Specify via dialog  padVal=0  spec=Output size  padNumOutRowsSpecMethod=User-specified  numOutRows=max(12, 6*modelDef.maxNumDelayedPoses)  padNumOutColsSpecMethod=User-specified  numOutCols=1  isVarDimsMode=off  padBeginning=0  padEnd=0  outSizeMode=User-specified  outSize=1  padSigAt=End  trunc_flag=None  roundingMode=Floor  overflowMode=off  truncOrWrapMode=Truncate  wrap_flag=None
      settings: SourceProductName=DSP System Toolbox  SourceProductBaseCode=DS
  Selector : Selector  NumberOfDimensions=2  InputPortWidth=3  IndexOptions=Starting index (dialog),Index vector (dialog)  Indices=1,1  OutputSizes=modelDef.numStates,modelDef.numStates
  Selector1 : Selector  NumberOfDimensions=2  InputPortWidth=3  IndexOptions=Starting index (dialog),Index vector (dialog)  Indices=modelDef.numStates+1,1  OutputSizes=6*modelDef.maxNumDelayedPoses,6*modelDef.maxNumDelayedPoses
  applyXstateErrors : Subsystem
  wires:
  For Each Subsystem/2(r_c_n_list) -> Data Store Write1/1
  For Each Subsystem/1(C_c_n_list) -> Data Store Write/1
  Data Store Read1/1 -> For Each Subsystem/3(r_c_n_list_in)
  Data Store Read/1 -> For Each Subsystem/2(C_c_n_list_in)
  Selector1/1 -> Pad/1
  Selector/1 -> applyXstateErrors/1(errorStateEstimates)
  errors/1 -> Selector/1, Selector1/1
  Pad/1 -> For Each Subsystem/1(delayedPoseCorrections)

== system VINS/measUpdate/absolutePoseUpdate/formMeasurementMatrix ==
  rows : Inport
  Assignment1 : Assignment  NumberOfDimensions=2  DiagnosticForDimensions=Warning  IndexOptions=Assign all,Index vector (port)  Indices=1,1  OutputSizes=1,1
  Constant1 : Constant  Value=zeros(6, 6*modelDef.maxNumDelayedPoses)  OutDataTypeStr=Inherit: Inherit via back propagation
  Constant2 : Constant  Value=eye(6)  OutDataTypeStr=Inherit: Inherit via back propagation
  Hx : Constant  Value=zeros(6, modelDef.numStates)  VectorParams1D=off  OutDataTypeStr=Inherit: Inherit via back propagation
  Matrix Concatenate : Concatenate  Mode=Multidimensional array  ConcatenateDimension=2
  Out1 : Outport
  wires:
  Constant2/1 -> Assignment1/2
  rows/1 -> Assignment1/3
  Assignment1/1 -> Matrix Concatenate/2
  Hx/1 -> Matrix Concatenate/1
  Matrix Concatenate/1 -> Out1/1
  Constant1/1 -> Assignment1/1

== system VINS/measUpdate/absolutePoseUpdate/get row indices ==
  idx : Inport
  Bias4 : Bias  Bias=(1:6)
  Constant3 : Constant  Value=uint8(1)
  Gain1 : Gain  Gain=6  OutDataTypeStr=Inherit: Same as input
  Sum2 : Sum  Inputs=|+-
  rows : Outport
  wires:
  Constant3/1 -> Sum2/2
  Sum2/1 -> Gain1/1
  Bias4/1 -> rows/1
  Gain1/1 -> Bias4/1
  idx/1 -> Sum2/1

== system VINS/measUpdate/absolutePoseUpdate/updateCovariance ==
  note: This repairs the covariance matrix by adding the smallest E matrix to it to make it positive definite.
  P : Inport
  H : Inport  Port=2
  K : Inport  Port=3
  R : Inport  Port=4
  Enable : EnablePort
  Data Store Write : DataStoreWrite  DataStoreName=Pxx
  Data Store Write1 : DataStoreWrite  DataStoreName=Pxc
  Data Store Write2 : DataStoreWrite  DataStoreName=Pcc
  Matrix 1-Norm1 : dspmtrx3/Matrix  1-Norm  roundingMode=Floor  overflowMode=off  outputDataTypeStr=Inherit: Same as accumulator  outputMin=[]  outputMax=[]  outputLastDataTypeStr=Inherit: Same as accumulator
      settings: SourceProductName=DSP System Toolbox  SourceProductBaseCode=DS
  Matrix Multiply : Product  Inputs=3  Multiplication=Matrix(*)
  Permute Dimensions1 : PermuteDimensions
  Scope3 : Scope
  Submatrix3 : dspmtrx3/Submatrix  RowSpan=Range of rows  RowStartMode=First  RowStartIndex=1  RowEndMode=Index  RowEndIndex=modelDef.numStates  ColSpan=Range of columns  ColStartMode=First  ColStartIndex=1  ColEndMode=Index  ColEndIndex=modelDef.numStates
  Submatrix4 : dspmtrx3/Submatrix  RowSpan=Range of rows  RowStartMode=First  RowStartIndex=1  RowEndMode=Index  RowEndIndex=modelDef.numStates  ColSpan=Range of columns  ColStartMode=Index  ColStartIndex=modelDef.numStates + 1  ColEndMode=Last  ColEndIndex=1
  Submatrix5 : dspmtrx3/Submatrix  RowSpan=Range of rows  RowStartMode=Index  RowStartIndex=modelDef.numStates + 1  RowEndMode=Last  RowEndIndex=modelDef.numStates  ColSpan=Range of columns  ColStartMode=Index  ColStartIndex=modelDef.numStates + 1  ColEndMode=Last  ColEndIndex=1
  josephCovarianceUpdate : MATLAB Function  TreatAsAtomicUnit=on
  modifiedCholesky : MATLAB Function  TreatAsAtomicUnit=on
  wires:
  josephCovarianceUpdate/1(Pplus) -> modifiedCholesky/1(G)
  P/1 -> josephCovarianceUpdate/1(P)
  Matrix 1-Norm1/1 -> Scope3/1
  Matrix Multiply/1 -> Submatrix5/1, Submatrix4/1, Submatrix3/1
  Submatrix5/1 -> Data Store Write2/1
  modifiedCholesky/2(D) -> Matrix Multiply/2
  modifiedCholesky/1(L) -> Permute Dimensions1/1, Matrix Multiply/1
  Submatrix3/1 -> Data Store Write/1
  Submatrix4/1 -> Data Store Write1/1
  modifiedCholesky/3(E) -> Matrix 1-Norm1/1
  Permute Dimensions1/1 -> Matrix Multiply/3
  R/1 -> josephCovarianceUpdate/4(R)
  H/1 -> josephCovarianceUpdate/3(H)
  K/1 -> josephCovarianceUpdate/2(K)

== system VINS/measUpdate/commanded reloc/DT convert2 ==
  In1 : Inport
  Data Store Read : DataStoreRead  DataStoreName=DataTypeRef
  Data Type Conversion Inherited : simulink/Signal Attributes/Data Type Conversion Inherited  ConvertRealWorld=Real World Value  DoSatur=off
      settings: SourceProductName=Simulink  SourceProductBaseCode=SL
  Out1 : Outport
  wires:
  In1/1 -> Data Type Conversion Inherited/2
  Data Store Read/1 -> Data Type Conversion Inherited/1
  Data Type Conversion Inherited/1 -> Out1/1

== system VINS/measUpdate/commanded reloc/DT convert3 ==
  In1 : Inport
  Data Store Read : DataStoreRead  DataStoreName=DataTypeRef
  Data Type Conversion Inherited : simulink/Signal Attributes/Data Type Conversion Inherited  ConvertRealWorld=Real World Value  DoSatur=off
      settings: SourceProductName=Simulink  SourceProductBaseCode=SL
  Out1 : Outport
  wires:
  Data Type Conversion Inherited/1 -> Out1/1
  Data Store Read/1 -> Data Type Conversion Inherited/1
  In1/1 -> Data Type Conversion Inherited/2

== system VINS/measUpdate/commanded reloc/setPosition1 ==
  r_nc_n : Inport
  yawChanged : Inport  Port=2
  Enable : EnablePort
  Constant10 : Constant  Value=0  OutDataTypeStr=Inherit: Inherit via back propagation
  Constant9 : Constant  Value=imuLocationMm  OutDataTypeStr=Inherit: Inherit via back propagation
  DT police3 : Subsystem  TreatAsAtomicUnit=on
  Data Store Read : DataStoreRead  DataStoreName=Cbn
  Data Store Write10 : DataStoreWrite  DataStoreName=distTravelled
  Data Store Write3 : DataStoreWrite  DataStoreName=rnav
  Gain : Gain  Gain=1/1000
  Matrix Multiply : Product  Multiplication=Matrix(*)
  Sum : Sum  Inputs=++|
  just to make sure yaw is updated first : Terminator
  wires:
  Sum/1 -> Data Store Write3/1  "r_nb_n"
  Matrix Multiply/1 -> Sum/1  "r_cb_n"
  Data Store Read/1 -> Matrix Multiply/1  "Ccn = Cbn"
  Constant9/1 -> Gain/1
  r_nc_n/1 -> Sum/2  "r_nc_n"
  Constant10/1 -> DT police3/1(In1), Data Store Write10/1
  Gain/1 -> Matrix Multiply/2  "r_cb_c"
  yawChanged/1 -> just to make sure yaw is updated first/1

== system VINS/measUpdate/commanded reloc/setYaw1 ==
  yaw : Inport
  Enable : EnablePort  ShowOutputPort=on
  Data Store Read : DataStoreRead  DataStoreName=Cbn
  Data Store Write3 : DataStoreWrite  DataStoreName=Cbn
  Demux : Demux  Outputs=3
  MATLAB Function3 : MATLAB Function  TreatAsAtomicUnit=on
  Mux : Mux  Inputs=3
  Permute Dimensions : PermuteDimensions
  Terminator : Terminator
  euler2dcm : MATLAB Function  TreatAsAtomicUnit=on
  yawChanged : Outport
  wires:
  Data Store Read/1 -> MATLAB Function3/1(Cbn)  "Ccn = Cbn"
  MATLAB Function3/1(eul) -> Demux/1
  Demux/1 -> Mux/1
  Demux/2 -> Mux/2
  yaw/1 -> Mux/3
  Demux/3 -> Terminator/1
  Mux/1 -> euler2dcm/1(eul_vect)
  euler2dcm/1(DCMnb) -> Permute Dimensions/1
  Permute Dimensions/1 -> Data Store Write3/1
  Enable/1 -> yawChanged/1

== system VINS/measUpdate/compass meas update/update the Cbn with the errors ==
  phi  rotation errors : Inport
  Data Store Read2 : DataStoreRead  DataStoreName=Cbn
  Data Store Write1 : DataStoreWrite  DataStoreName=Cbn
  MATLAB Function : MATLAB Function  TreatAsAtomicUnit=on
  Product2 : Product  Multiplication=Matrix(*)
  Sum : Sum  Inputs=++|
  re-orthonormalization : Subsystem  TreatAsAtomicUnit=on
  wires:
  MATLAB Function/1(res) -> Product2/1  "[phi X]"
  Product2/1 -> Sum/1
  Sum/1 -> re-orthonormalization/1(In1)
  phi  rotation errors/1 -> MATLAB Function/1(inp_vr)
  Data Store Read2/1 -> Product2/2, Sum/2
  re-orthonormalization/1(Out1) -> Data Store Write1/1

== system VINS/measUpdate/get pose indices/almostEqual ==
  In1 : Inport
  In2 : Inport  Port=2
  Abs : Abs
  Constant2 : Constant  Value=timeMatchThreshold  OutDataTypeStr=Inherit: Inherit via back propagation
  Relational Operator : RelationalOperator  Operator=<=  OutDataTypeStr=boolean  RndMeth=Simplest
  Sum2 : Sum  Inputs=+-
  Out1 : Outport
  wires:
  Constant2/1 -> Relational Operator/2
  Abs/1 -> Relational Operator/1
  Sum2/1 -> Abs/1
  In1/1 -> Sum2/1
  In2/1 -> Sum2/2
  Relational Operator/1 -> Out1/1

== system VINS/measUpdate/get pose indices/almostEqual1 ==
  In1 : Inport
  In2 : Inport  Port=2
  Abs : Abs
  Constant2 : Constant  Value=timeMatchThreshold  OutDataTypeStr=Inherit: Inherit via back propagation
  Relational Operator : RelationalOperator  Operator=<=  OutDataTypeStr=boolean  RndMeth=Simplest
  Sum2 : Sum  Inputs=+-
  Out1 : Outport
  wires:
  Relational Operator/1 -> Out1/1
  In2/1 -> Sum2/2
  In1/1 -> Sum2/1
  Sum2/1 -> Abs/1
  Abs/1 -> Relational Operator/1
  Constant2/1 -> Relational Operator/2

== system VINS/measUpdate/get pose indices1/almostEqual ==
  In1 : Inport
  In2 : Inport  Port=2
  Abs : Abs
  Constant2 : Constant  Value=timeMatchThreshold  OutDataTypeStr=Inherit: Inherit via back propagation
  Relational Operator : RelationalOperator  Operator=<=  OutDataTypeStr=boolean  RndMeth=Simplest
  Sum2 : Sum  Inputs=+-
  Out1 : Outport
  wires:
  Constant2/1 -> Relational Operator/2
  Abs/1 -> Relational Operator/1
  Sum2/1 -> Abs/1
  In1/1 -> Sum2/1
  In2/1 -> Sum2/2
  Relational Operator/1 -> Out1/1

== system VINS/measUpdate/gravity meas update/update the Cbn and b_g with the errors ==
  " error state estimates" : Inport
  Data Store Read1 : DataStoreRead  DataStoreName=dw
  Data Store Read2 : DataStoreRead  DataStoreName=Cbn
  Data Store Read3 : DataStoreRead  DataStoreName=rnav
  Data Store Read4 : DataStoreRead  DataStoreName=vnav
  Data Store Read5 : DataStoreRead  DataStoreName=df
  Data Store Read6 : DataStoreRead  DataStoreName=Macc
  Data Store Read7 : DataStoreRead  DataStoreName=Mgyr
  Data Store Write1 : DataStoreWrite  DataStoreName=Cbn
  Data Store Write2 : DataStoreWrite  DataStoreName=dw
  Data Store Write3 : DataStoreWrite  DataStoreName=rnav
  Data Store Write4 : DataStoreWrite  DataStoreName=vnav
  Data Store Write5 : DataStoreWrite  DataStoreName=df
  Data Store Write6 : DataStoreWrite  DataStoreName=Macc
  Data Store Write7 : DataStoreWrite  DataStoreName=Mgyr
  MATLAB Function : MATLAB Function  TreatAsAtomicUnit=on
  Multiport Selector : dspindex/Multiport Selector  rowsOrCols=Rows  idxCellArray={ 1:3, 4:6, 7:9, 10:12, 13:15, 16:24, 25:33 }  idxErrMode=Clip Index
  Product2 : Product  Multiplication=Matrix(*)
  Reshape : Reshape  OutputDimensionality=Customize  OutputDimensions=[3,3]
  Reshape1 : Reshape  OutputDimensionality=Customize  OutputDimensions=[3,3]
  Sum{,1..6} (7 alike) : Sum  Inputs=++|
  re-orthonormalization : Subsystem  TreatAsAtomicUnit=on
  wires:
  Reshape1/1 -> Sum6/1
  Multiport Selector/7 -> Reshape1/1
  Reshape/1 -> Sum5/1
  Multiport Selector/6 -> Reshape/1
  Data Store Read7/1 -> Sum6/2
  Sum6/1 -> Data Store Write7/1
  Sum5/1 -> Data Store Write6/1
  Data Store Read6/1 -> Sum5/2
  Multiport Selector/5 -> Sum4/1
  Data Store Read5/1 -> Sum4/2
  Sum4/1 -> Data Store Write5/1
  Multiport Selector/4 -> Sum3/1
  Multiport Selector/3 -> Sum2/1
  Sum3/1 -> Data Store Write4/1
  Data Store Read4/1 -> Sum3/2
  Data Store Read3/1 -> Sum2/2
  Sum2/1 -> Data Store Write3/1
  " error state estimates"/1 -> Multiport Selector/1
  Multiport Selector/2 -> Sum1/1  "gyro bias errors"
  Sum1/1 -> Data Store Write2/1
  Data Store Read1/1 -> Sum1/2
  Multiport Selector/1 -> MATLAB Function/1(inp_vr)  "phi rotation errors"
  re-orthonormalization/1(Out1) -> Data Store Write1/1
  Data Store Read2/1 -> Sum/2, Product2/2
  Sum/1 -> re-orthonormalization/1(In1)
  Product2/1 -> Sum/1
  MATLAB Function/1(res) -> Product2/1  "[phi X]"

== system VINS/measUpdate/modeController/set useRpus = true ==
  Enable : EnablePort
  Constant : Constant  Value=true
  Data Store Write : DataStoreWrite  DataStoreName=useRpus
  wires:
  Constant/1 -> Data Store Write/1

== system VINS/measUpdate/opticalValid/DT convert1 ==
  In1 : Inport
  Data Store Read : DataStoreRead  DataStoreName=DataTypeRef
  Data Type Conversion Inherited : simulink/Signal Attributes/Data Type Conversion Inherited  ConvertRealWorld=Real World Value  DoSatur=off
      settings: SourceProductName=Simulink  SourceProductBaseCode=SL
  Out1 : Outport
  wires:
  In1/1 -> Data Type Conversion Inherited/2
  Data Store Read/1 -> Data Type Conversion Inherited/1
  Data Type Conversion Inherited/1 -> Out1/1
